simulink model "LdLq_Constant_Feedforward_1000"  (R2020a)
settings: Solver=ode4  StartTime=0.0  StopTime=10*T  FixedStep=1e-6  RelTol=1e-3  EnableMultiTasking=on
values from neighbouring files (symbols this model uses):
  Beta = effydata(i, 4)    [auto_effymap_real_current_idiq.m]
  Imag = effydata(i, 3)    [auto_effymap_real_current_idiq.m]
  Kad = 1/Kpd    [auto_effymap_real_current_idiq.m]
  Kaq = 1/Kpq    [auto_effymap_real_current_idiq.m]
  Kid = R*wc*100    (= 723.24329)    [auto_effymap_real_current_idiq.m]
  Kiq = R*wc*100    (= 723.24329)    [auto_effymap_real_current_idiq.m]
  Kpd = Ld*wc*10    [auto_effymap_real_current_idiq.m]
  Kpq = Lq*wc*10    [auto_effymap_real_current_idiq.m]
  Lamda_f = mean(lamda_d)    [auto_effymap_real_current_idiq.m]
  Ld = (lambda_d-Lamda_f)/id    [auto_effymap_real_current_idiq.m]
  Lq = lambda_q/iq    [auto_effymap_real_current_idiq.m]
  Np = 8    [auto_effymap_real_current_idiq.m]
  R = 0.013149878    [auto_effymap_real_current_idiq.m]
  rpm = Input.base_rpm    [Run_for_emf.m]    (also in Run_for_emf_skew.m; Run_for_lamda.m; Run_for_lamda_skew.m; Run_for_loss.m = Eff_Map_i(1))
  sf = 5500    [auto_effymap_real_current_idiq.m]
  Vdc = 320    [auto_effymap_real_current_idiq.m]
libraries: powerlib x17, simulink x4
settings Model: Creator=SONBK  LastModifiedBy=JSB-PC
settings DataIOCC: LimitDataPoints=on  SaveFormat=Array  SignalLoggingSaveFormat=ModelDataLogs  ReturnWorkspaceOutputs=off
settings OptimizationCC: ExpressionDepthLimit=2147483647  LifeSpan=inf
settings DebuggingCC: UnderspecifiedInitializationDetection=Classic  MergeDetectMultiDrivingBlocksExec=none  SolverPrmCheckMsg=warning  FcnCallInpInsideContextMsg=warning  AllowSymbolicDim=off  StateNameClashWarn=warning  SFUnexpectedBacktrackingDiag=warning  SFNoUnconditionalDefaultTransitionDiag=warning  SFExecutionAtInitializationDiag=none  ArithmeticOperatorsInVariantConditions=warning
settings HardwareCC: ProdBitPerPointer=32  ProdBitPerSizeT=32  ProdBitPerPtrDiffT=32  ProdLargestAtomicFloat=None  ProdIntDivRoundTo=Undefined  ProdEndianess=Unspecified  ProdWordSize=32  ProdHWDeviceType=32-bit Generic
settings ModelReferenceCC: PropagateSignalLabelsOutOfModel=off
settings SFSimCC: SimUseLocalCustomCode=off  CustomCodeUndefinedFunction=UseInterfaceOnly
settings RTWCC: RTWUseLocalCustomCode=off
settings CodeAppCC: StateflowObjectComments=on
settings GRTTargetCC: TargetLangStandard=C89/C90 (ANSI)  CombineOutputUpdateFcns=off  GRTInterface=on
settings ConfigComp: CovMetricSettings=dw  CovHtmlReporting=on  CovSaveCumulativeToWorkspaceVar=on  CovSaveSingleToWorkspaceVar=on  CovExternalEMLEnable=off
settings SimscapeCC: SimscapeNormalizeSystem=off

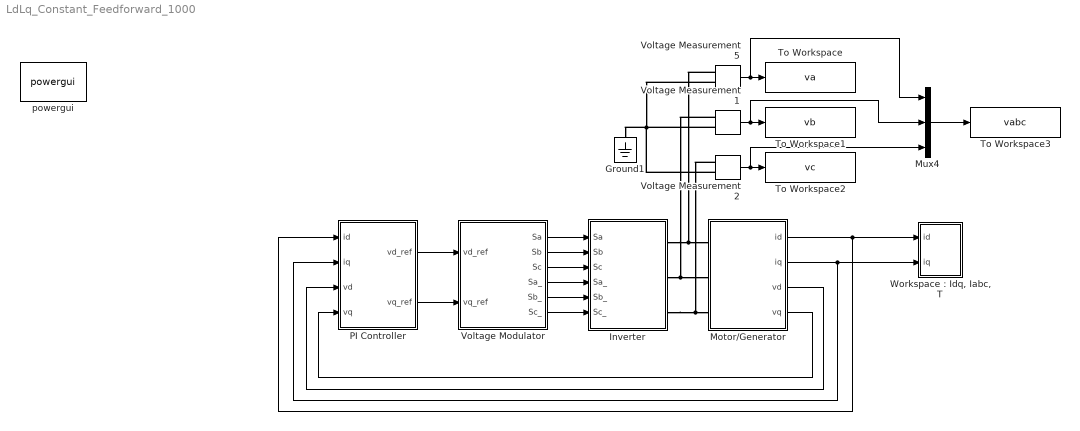
== system LdLq_Constant_Feedforward_1000 ==
  Ground1 : powerlib/Elements/Ground  LConnTagsString=a
  Inverter : Subsystem
  Motor/Generator : Subsystem
  Mux4 : Mux  Inputs=3
  PI Controller : Subsystem
  To Workspace : ToWorkspace  VariableName=va  SampleTime=-1
  To Workspace1 : ToWorkspace  VariableName=vb  SampleTime=-1
  To Workspace2 : ToWorkspace  VariableName=vc  SampleTime=-1
  To Workspace3 : ToWorkspace  VariableName=vabc  SampleTime=-1
  Voltage Measurement1 : powerlib/Measurements/Voltage Measurement  PhasorSimulation=off  OutputType=Complex  PSBequivalent=0
  Voltage Measurement2 : powerlib/Measurements/Voltage Measurement  PhasorSimulation=off  OutputType=Complex  PSBequivalent=0
  Voltage Measurement5 : powerlib/Measurements/Voltage Measurement  PhasorSimulation=off  OutputType=Complex  PSBequivalent=0
  Voltage Modulator : Subsystem
  "Workspace : Idq, Iabc, T" : Subsystem
  powergui : powerlib/powergui  Priority=1  SimulationMode=Continuous  SampleTime=50e-6  frequency=60  Iterations=50  frequencyindice=0  Pbase=100e6  ErrMax=1e-4  UnitsV=kV  UnitsW=MW  buscounter=0  FunctionMessages=off  echomessages=off  EnableUseOfTLC=off  CurrentSourceSwitches=off  DisableSnubberDevices=off  DisableRonSwitches=off  DisableVfSwitches=off  DisplayEquations=off  AutomaticDiscreteSolvers=off  SolverType=Tustin/Backward Euler (TBE)  Interpol=off  ExternalGateDelay=off  methode=off  Ts=10  x0status=blocks  SPID=on  SwTol=0  HookPort=off  NonlinearTolerance=1e-4  nMaxIteration=100  ContinueOnMaxIteration=off  RestoreLinks=warning  ResistiveCurrentMeasurement=off  Frange=[0:2:500]  Ylog=off  Xlog=on  ShowGrid=off  save=off  variable=ZData  structure=0  ZoomFFT=off  StartTime=0.0  cycles=1  DisplayStyle=1  fundamental=60  FreqAxis=off  MaxFrequency=1000  frequencyindicesteady=1  RmsSteady=1  display=off
  wires:
  Voltage Modulator/1(Sa) -> Inverter/1(Sa)
  Voltage Modulator/2(Sb) -> Inverter/2(Sb)
  Voltage Modulator/3(Sc) -> Inverter/3(Sc)
  Voltage Modulator/4(Sa_) -> Inverter/4(Sa_)
  Voltage Modulator/5(Sb_) -> Inverter/5(Sb_)
  Voltage Modulator/6(Sc_) -> Inverter/6(Sc_)
  Motor/Generator/2(iq) -> PI Controller/2(iq), "Workspace : Idq, Iabc, T"/2(iq)
  Motor/Generator/1(id) -> "Workspace : Idq, Iabc, T"/1(id), PI Controller/1(id)
  Motor/Generator/3(vd) -> PI Controller/3(vd)
  Motor/Generator/4(vq) -> PI Controller/4(vq)
  PI Controller/1(vd_ref) -> Voltage Modulator/1(vd_ref)
  PI Controller/2(vq_ref) -> Voltage Modulator/2(vq_ref)
  Voltage Measurement5/1 -> Mux4/1, To Workspace/1
  Voltage Measurement1/1 -> Mux4/2, To Workspace1/1
  Voltage Measurement2/1 -> Mux4/3, To Workspace2/1
  Mux4/1 -> To Workspace3/1
  connections:
  Inverter/RConn1 -- Voltage Measurement5/LConn1 -- Motor/Generator/LConn1
  Inverter/RConn2 -- Voltage Measurement1/LConn1 -- Motor/Generator/LConn2
  Inverter/RConn3 -- Voltage Measurement2/LConn1 -- Motor/Generator/LConn3
  Voltage Measurement1/LConn2 -- Ground1/LConn1 -- Voltage Measurement5/LConn2 -- Voltage Measurement2/LConn2

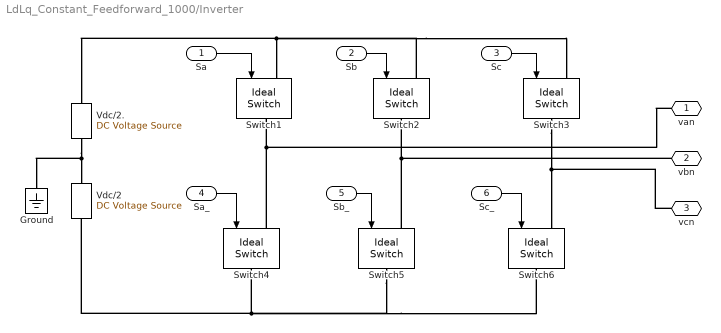
== system LdLq_Constant_Feedforward_1000/Inverter ==
  Sa : Inport
  Sb : Inport  Port=2
  Sc : Inport  Port=3
  Sa_ : Inport  Port=4
  Sb_ : Inport  Port=5
  Sc_ : Inport  Port=6
  Ground : powerlib/Elements/Ground  LConnTagsString=a
  Switch{1..6} (6 alike) : powerlib/Power Electronics/Ideal Switch  Ron=0.001  Lon=0  IC=0  Rs=1e5  Cs=inf  Measurements=off
      settings: AttributesFormatString=\n
  Vdc/2 : powerlib/Electrical Sources/DC Voltage Source  Amplitude=Vdc/2  Measurements=None
  Vdc/2. : powerlib/Electrical Sources/DC Voltage Source  Amplitude=Vdc/2  Measurements=None
  van : PMIOPort  Side=Right
  vbn : PMIOPort  Port=2  Side=Right
  vcn : PMIOPort  Port=3  Side=Right
  wires:
  Sb/1 -> Switch2/1
  Sc/1 -> Switch3/1
  Sa/1 -> Switch1/1
  Sb_/1 -> Switch5/1
  Sa_/1 -> Switch4/1
  Sc_/1 -> Switch6/1
  connections:
  Switch3/LConn1 -- Switch2/LConn1 -- Vdc/2./RConn1 -- Switch1/LConn1
  Switch3/RConn1 -- Switch6/LConn1 -- vcn/RConn1
  Switch6/RConn1 -- Switch5/RConn1 -- Switch4/RConn1 -- Vdc/2/LConn1
  Vdc/2./LConn1 -- Vdc/2/RConn1 -- Ground/LConn1
  Switch5/LConn1 -- Switch2/RConn1 -- vbn/RConn1
  Switch4/LConn1 -- van/RConn1 -- Switch1/RConn1

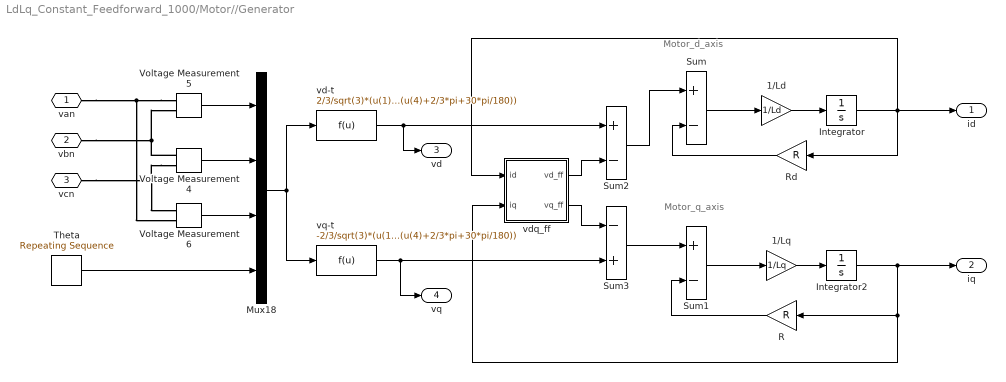
== system LdLq_Constant_Feedforward_1000/Motor//Generator ==
  note: Motor_q_axis
  note: Motor_d_axis
  1/Ld : Gain  Gain=1/Ld
  1/Lq : Gain  Gain=1/Lq
  Integrator : Integrator
  Integrator2 : Integrator
  Mux18 : Mux
  R : Gain  Gain=R
  Rd : Gain  Gain=R
  Sum : Sum  Inputs=+-
  Sum1 : Sum  Inputs=+-
  Sum2 : Sum  Inputs=+-
  Sum3 : Sum  Inputs=-+
  Theta : simulink/Sources/Repeating Sequence  rep_seq_t=[0 1/(rpm/60*Np/2)]  rep_seq_y=[0 2*pi()]
  Voltage Measurement4 : powerlib/Measurements/Voltage Measurement  PhasorSimulation=off  OutputType=Complex  PSBequivalent=0
  Voltage Measurement5 : powerlib/Measurements/Voltage Measurement  PhasorSimulation=off  OutputType=Complex  PSBequivalent=0
  Voltage Measurement6 : powerlib/Measurements/Voltage Measurement  PhasorSimulation=off  OutputType=Complex  PSBequivalent=0
  vd-t : Fcn  Expr=2/3/sqrt(3)*(u(1)*cos(u(4)+30*pi/180)+u(2)*cos(u(4)-2/3*pi+30*pi/180)+u(3)*cos(u(4)+2/3*pi+30*pi/180))
  vdq_ff : Subsystem
  vq-t : Fcn  Expr=-2/3/sqrt(3)*(u(1)*sin(u(4)+30*pi/180)+u(2)*sin(u(4)-2/3*pi+30*pi/180)+u(3)*sin(u(4)+2/3*pi+30*pi/180))
  van : PMIOPort  Side=Left
  vbn : PMIOPort  Port=2  Side=Left
  vcn : PMIOPort  Port=3  Side=Left
  id : Outport
  iq : Outport  Port=2
  vd : Outport  Port=3
  vq : Outport  Port=4
  wires:
  Voltage Measurement4/1 -> Mux18/2
  Voltage Measurement5/1 -> Mux18/1
  Mux18/1 -> vq-t/1, vd-t/1
  Voltage Measurement6/1 -> Mux18/3
  Theta/1 -> Mux18/4
  vd-t/1 -> Sum2/1, vd/1
  Rd/1 -> Sum/2
  Integrator2/1 -> vdq_ff/2(iq), R/1, iq/1
  1/Ld/1 -> Integrator/1
  Sum/1 -> 1/Ld/1
  Integrator/1 -> vdq_ff/1(id), id/1, Rd/1
  Sum1/1 -> 1/Lq/1
  vq-t/1 -> Sum3/2, vq/1
  R/1 -> Sum1/2
  1/Lq/1 -> Integrator2/1
  Sum2/1 -> Sum/1
  Sum3/1 -> Sum1/1
  vdq_ff/1(vd_ff) -> Sum2/2
  vdq_ff/2(vq_ff) -> Sum3/1
  connections:
  Voltage Measurement4/LConn2 -- vcn/RConn1 -- Voltage Measurement6/LConn1
  Voltage Measurement5/LConn1 -- van/RConn1 -- Voltage Measurement6/LConn2
  Voltage Measurement4/LConn1 -- vbn/RConn1 -- Voltage Measurement5/LConn2

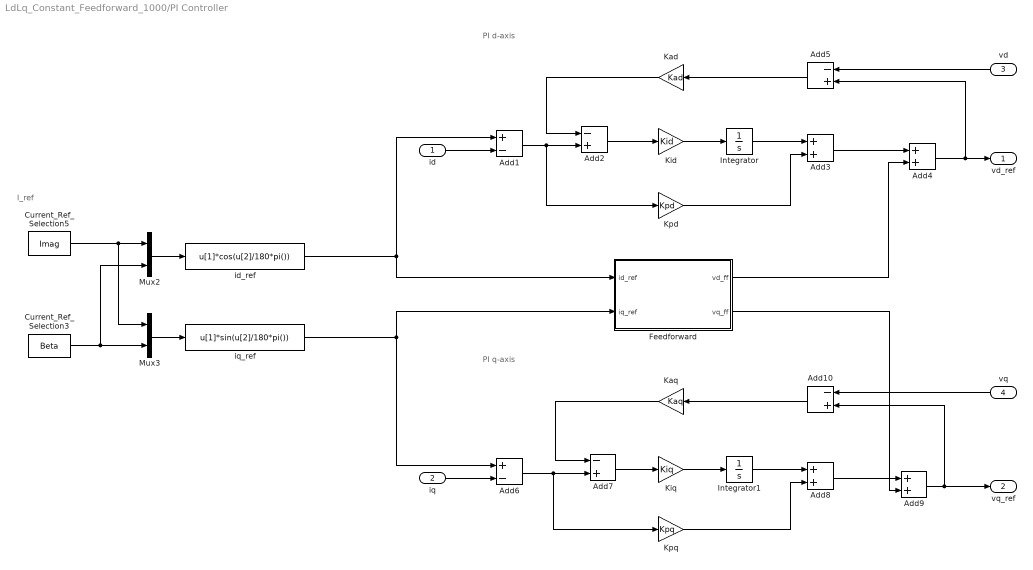
== system LdLq_Constant_Feedforward_1000/PI Controller ==
  note: I_ref
  note: PI q-axis
  note: PI d-axis
  id : Inport
  iq : Inport  Port=2
  vd : Inport  Port=3
  vq : Inport  Port=4
  Add1 : Sum  Inputs=+-
  Add{2,5,7,10} (4 alike) : Sum  Inputs=-+
  Add{3..4,8..9} (4 alike) : Sum
  Add6 : Sum  Inputs=+-
  Current_Ref_Selection3 : Constant  DisableCoverage=on  Value=Beta
  Current_Ref_Selection5 : Constant  Description=Ipk  DisableCoverage=on  Value=Imag
  Feedforward : Subsystem
  Integrator : Integrator
  Integrator1 : Integrator
  Kad : Gain  Gain=Kad
  Kaq : Gain  Gain=Kaq
  Kid : Gain  Gain=Kid
  Kiq : Gain  Gain=Kiq
  Kpd : Gain  Gain=Kpd
  Kpq : Gain  Gain=Kpq
  Mux2 : Mux  Inputs=2
  Mux3 : Mux  Inputs=2
  id_ref : Fcn  Expr=u[1]*cos(u[2]/180*pi())
  iq_ref : Fcn  Expr=u[1]*sin(u[2]/180*pi())
  vd_ref : Outport
  vq_ref : Outport  Port=2
  wires:
  Add9/1 -> Add10/2, vq_ref/1
  Add4/1 -> Add5/2, vd_ref/1
  vq/1 -> Add10/1
  vd/1 -> Add5/1
  Add10/1 -> Kaq/1
  Kaq/1 -> Add7/1
  Add7/1 -> Kiq/1
  Kad/1 -> Add2/1
  Add1/1 -> Kpd/1, Add2/2
  Add2/1 -> Kid/1
  Add5/1 -> Kad/1
  iq_ref/1 -> Add6/1, Feedforward/2(iq_ref)
  Kiq/1 -> Integrator1/1
  Kpq/1 -> Add8/2
  Integrator1/1 -> Add8/1
  Add6/1 -> Add7/2, Kpq/1
  id_ref/1 -> Feedforward/1(id_ref), Add1/1
  Add3/1 -> Add4/1
  Kid/1 -> Integrator/1
  Kpd/1 -> Add3/2
  Integrator/1 -> Add3/1
  Current_Ref_Selection5/1 -> Mux2/1, Mux3/1
  Current_Ref_Selection3/1 -> Mux3/2, Mux2/2
  Mux3/1 -> iq_ref/1
  Mux2/1 -> id_ref/1
  iq/1 -> Add6/2
  id/1 -> Add1/2
  Add8/1 -> Add9/1
  Feedforward/2(vq_ff) -> Add9/2
  Feedforward/1(vd_ff) -> Add4/2

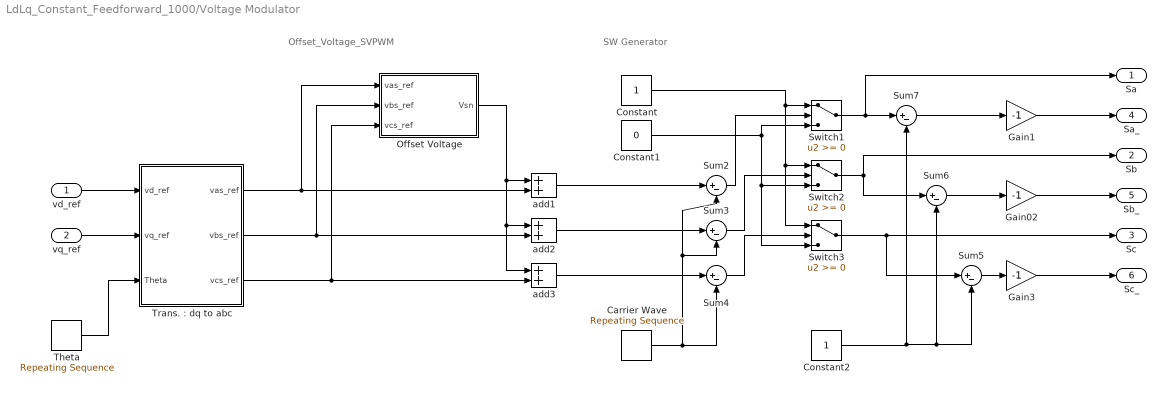
== system LdLq_Constant_Feedforward_1000/Voltage Modulator ==
  note: SW Generator
  note: Offset_Voltage_SVPWM
  vd_ref : Inport
  vq_ref : Inport  Port=2
  Carrier Wave : simulink/Sources/Repeating Sequence  rep_seq_t=[0 0.5/sf 1/sf]  rep_seq_y=[-Vdc/2 Vdc/2 -Vdc/2]
  Constant : Constant
  Constant1 : Constant  Value=0
  Constant2 : Constant
  Gain02 : Gain  Gain=-1  SaturateOnIntegerOverflow=on  OutDataTypeStr=Inherit: Same as input  ParamDataTypeStr=Inherit: Same as input
  Gain1 : Gain  Gain=-1  SaturateOnIntegerOverflow=on  OutDataTypeStr=Inherit: Same as input  ParamDataTypeStr=Inherit: Same as input
  Gain3 : Gain  Gain=-1  SaturateOnIntegerOverflow=on  OutDataTypeStr=Inherit: Same as input  ParamDataTypeStr=Inherit: Same as input
  Offset Voltage : Subsystem
  Sum{2..7} (6 alike) : Sum  Inputs=|+-  SaturateOnIntegerOverflow=on
  Switch1 : Switch  SaturateOnIntegerOverflow=on
  Switch2 : Switch  SaturateOnIntegerOverflow=on
  Switch3 : Switch  SaturateOnIntegerOverflow=on
  Theta : simulink/Sources/Repeating Sequence  rep_seq_t=[0 1/(rpm/60*Np/2)]  rep_seq_y=[0 2*pi()]
  "Trans. : dq to abc" : Subsystem
  add1 : Sum  Inputs=2  InputSameDT=on  SaturateOnIntegerOverflow=on  OutDataTypeStr=Inherit: Same as first input
  add2 : Sum  Inputs=2  InputSameDT=on  SaturateOnIntegerOverflow=on  OutDataTypeStr=Inherit: Same as first input
  add3 : Sum  Inputs=2  InputSameDT=on  SaturateOnIntegerOverflow=on  OutDataTypeStr=Inherit: Same as first input
  Sa : Outport
  Sb : Outport  Port=2
  Sc : Outport  Port=3
  Sa_ : Outport  Port=4
  Sb_ : Outport  Port=5
  Sc_ : Outport  Port=6
  wires:
  Gain1/1 -> Sa_/1
  Gain02/1 -> Sb_/1
  Switch3/1 -> Sum5/1, Sc/1
  Switch1/1 -> Sum7/1, Sa/1
  Switch2/1 -> Sb/1, Sum6/1
  Gain3/1 -> Sc_/1
  add3/1 -> Sum4/1
  Sum7/1 -> Gain1/1
  Sum5/1 -> Gain3/1
  Sum6/1 -> Gain02/1
  Constant2/1 -> Sum6/2, Sum5/2, Sum7/2
  Sum2/1 -> Switch1/2
  Constant1/1 -> Switch1/3, Switch3/3, Switch2/3
  Constant/1 -> Switch3/1, Switch2/1, Switch1/1
  Sum4/1 -> Switch3/2
  Sum3/1 -> Switch2/2
  add1/1 -> Sum2/1
  add2/1 -> Sum3/1
  Carrier Wave/1 -> Sum2/2, Sum3/2, Sum4/2
  "Trans. : dq to abc"/2(vbs_ref) -> Offset Voltage/2(vbs_ref), add2/2
  "Trans. : dq to abc"/1(vas_ref) -> Offset Voltage/1(vas_ref), add1/2
  "Trans. : dq to abc"/3(vcs_ref) -> Offset Voltage/3(vcs_ref), add3/2
  vd_ref/1 -> "Trans. : dq to abc"/1(vd_ref)
  vq_ref/1 -> "Trans. : dq to abc"/2(vq_ref)
  Theta/1 -> "Trans. : dq to abc"/3(Theta)
  Offset Voltage/1(Vsn) -> add3/1, add2/1, add1/1

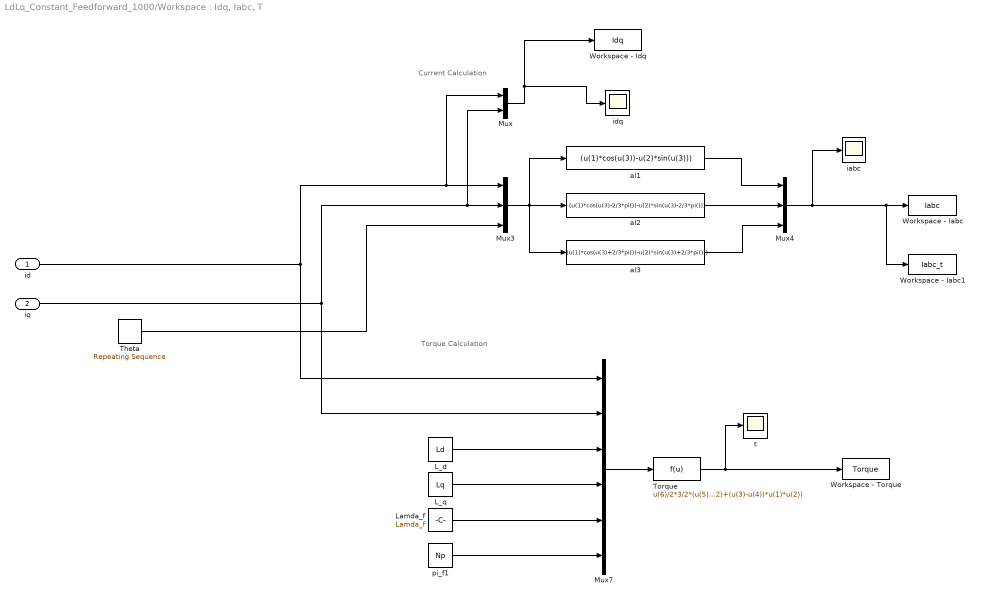
== system LdLq_Constant_Feedforward_1000/Workspace : Idq, Iabc, T ==
  note: Torque Calculation
  note: Current Calculation
  id : Inport
  iq : Inport  Port=2
  L_d : Constant  Value=Ld
  L_q : Constant  Value=Lq
  Lamda_f : Constant  Value=Lamda_f
  Mux : Mux  Inputs=2
  Mux3 : Mux  Inputs=3
  Mux4 : Mux  Inputs=3
  Mux7 : Mux  Inputs=6
  Theta : simulink/Sources/Repeating Sequence  rep_seq_t=[0 1/(rpm/60*Np/2)]  rep_seq_y=[0 2*pi()]
  Torque : Fcn  Expr=u(6)/2*3/2*(u(5)*u(2)+(u(3)-u(4))*u(1)*u(2))
  Workspace - Iabc : ToWorkspace  VariableName=Iabc  SampleTime=-1
  Workspace - Iabc1 : ToWorkspace  VariableName=Iabc_t  SaveFormat=Structure With Time  SampleTime=-1
  Workspace - Idq : ToWorkspace  VariableName=Idq  SampleTime=-1
  Workspace - Torque : ToWorkspace  VariableName=Torque  SampleTime=-1
  al1 : Fcn  Expr=(u(1)*cos(u(3))-u(2)*sin(u(3)))
  al2 : Fcn  Expr=(u(1)*cos(u(3)-2/3*pi())-u(2)*sin(u(3)-2/3*pi()))
  al3 : Fcn  Expr=(u(1)*cos(u(3)+2/3*pi())-u(2)*sin(u(3)+2/3*pi()))
  iabc : Scope
  idq : Scope
  pi_f1 : Constant  Value=Np
  t : Scope
  wires:
  Torque/1 -> Workspace - Torque/1, t/1
  Mux/1 -> Workspace - Idq/1, idq/1
  Mux4/1 -> Workspace - Iabc1/1, Workspace - Iabc/1, iabc/1
  al3/1 -> Mux4/3
  al2/1 -> Mux4/2
  Theta/1 -> Mux3/3
  al1/1 -> Mux4/1
  Lamda_f/1 -> Mux7/5
  Mux3/1 -> al3/1, al1/1, al2/1
  pi_f1/1 -> Mux7/6
  Mux7/1 -> Torque/1
  L_q/1 -> Mux7/4
  iq/1 -> Mux7/2, Mux3/2, Mux/2
  L_d/1 -> Mux7/3
  id/1 -> Mux7/1, Mux/1, Mux3/1

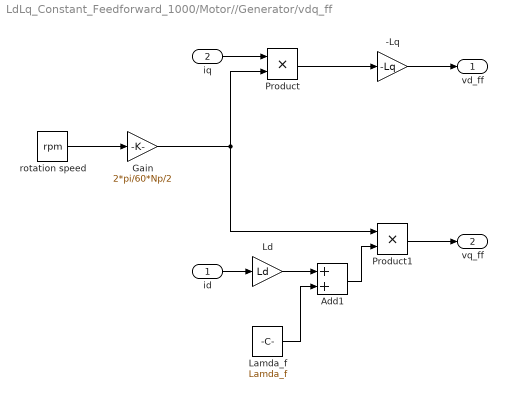
== system LdLq_Constant_Feedforward_1000/Motor//Generator/vdq_ff ==
  id : Inport
  iq : Inport  Port=2
  -Lq : Gain  Gain=-Lq
  Add1 : Sum
  Gain : Gain  Gain=2*pi/60*Np/2  SaturateOnIntegerOverflow=on  OutDataTypeStr=Inherit: Same as input  ParamDataTypeStr=Inherit: Same as input
  Lamda_f : Constant  Value=Lamda_f
  Ld : Gain  Gain=Ld
  Product : Product  RndMeth=Zero
  Product1 : Product  RndMeth=Zero
  rotation speed : Constant  Value=rpm
  vd_ff : Outport
  vq_ff : Outport  Port=2
  wires:
  Product/1 -> -Lq/1
  rotation speed/1 -> Gain/1
  Ld/1 -> Add1/1
  Gain/1 -> Product1/1, Product/2
  -Lq/1 -> vd_ff/1
  Add1/1 -> Product1/2
  Product1/1 -> vq_ff/1
  Lamda_f/1 -> Add1/2
  id/1 -> Ld/1
  iq/1 -> Product/1

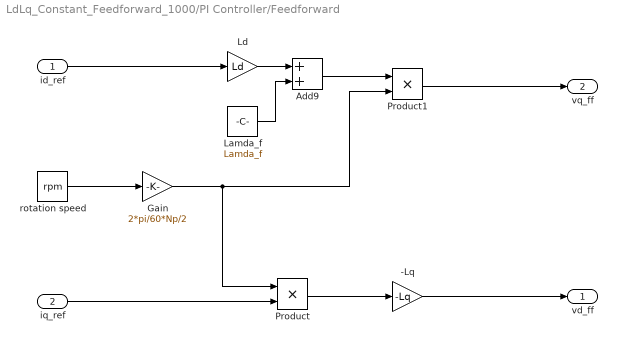
== system LdLq_Constant_Feedforward_1000/PI Controller/Feedforward ==
  id_ref : Inport
  iq_ref : Inport  Port=2
  -Lq : Gain  Gain=-Lq
  Add9 : Sum
  Gain : Gain  Gain=2*pi/60*Np/2  SaturateOnIntegerOverflow=on  OutDataTypeStr=Inherit: Same as input  ParamDataTypeStr=Inherit: Same as input
  Lamda_f : Constant  Value=Lamda_f
  Ld : Gain  Gain=Ld
  Product : Product  RndMeth=Zero
  Product1 : Product  RndMeth=Zero
  rotation speed : Constant  Value=rpm
  vd_ff : Outport
  vq_ff : Outport  Port=2
  wires:
  rotation speed/1 -> Gain/1
  Product1/1 -> vq_ff/1
  Ld/1 -> Add9/1
  -Lq/1 -> vd_ff/1
  Gain/1 -> Product/1, Product1/2
  Lamda_f/1 -> Add9/2
  Product/1 -> -Lq/1
  Add9/1 -> Product1/1
  id_ref/1 -> Ld/1
  iq_ref/1 -> Product/2

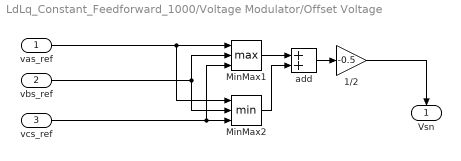
== system LdLq_Constant_Feedforward_1000/Voltage Modulator/Offset Voltage ==
  vas_ref : Inport
  vbs_ref : Inport  Port=2
  vcs_ref : Inport  Port=3
  1/2 : Gain  Gain=-0.5
  MinMax1 : MinMax  Function=max  Inputs=3
  MinMax2 : MinMax  Inputs=3
  add : Sum  Inputs=2  InputSameDT=on  SaturateOnIntegerOverflow=on  OutDataTypeStr=Inherit: Same as first input
  Vsn : Outport
  wires:
  1/2/1 -> Vsn/1
  add/1 -> 1/2/1
  MinMax2/1 -> add/2
  MinMax1/1 -> add/1
  vcs_ref/1 -> MinMax2/3, MinMax1/3
  vbs_ref/1 -> MinMax2/2, MinMax1/2
  vas_ref/1 -> MinMax2/1, MinMax1/1

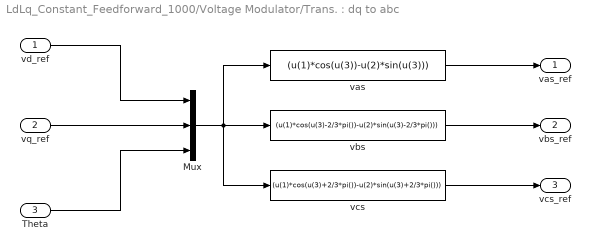
== system LdLq_Constant_Feedforward_1000/Voltage Modulator/Trans. : dq to abc ==
  vd_ref : Inport
  vq_ref : Inport  Port=2
  Theta : Inport  Port=3
  Mux : Mux  Inputs=3
  vas : Fcn  Expr=(u(1)*cos(u(3))-u(2)*sin(u(3)))
  vbs : Fcn  Expr=(u(1)*cos(u(3)-2/3*pi())-u(2)*sin(u(3)-2/3*pi()))
  vcs : Fcn  Expr=(u(1)*cos(u(3)+2/3*pi())-u(2)*sin(u(3)+2/3*pi()))
  vas_ref : Outport
  vbs_ref : Outport  Port=2
  vcs_ref : Outport  Port=3
  wires:
  vq_ref/1 -> Mux/2
  vd_ref/1 -> Mux/1
  vas/1 -> vas_ref/1
  vbs/1 -> vbs_ref/1
  vcs/1 -> vcs_ref/1
  Mux/1 -> vcs/1, vas/1, vbs/1
  Theta/1 -> Mux/3
